simulink model "sarzni_reaktor1_2"  (R2020b)
settings: Solver=VariableStepAuto  StartTime=0.0  StopTime=tSim  RelTol=1e-3
values from neighbouring files (symbols this model uses):
  T_ref = 50    [reactortest.m]
libraries: pid_lib x2, reaktor x1
settings Model: Creator=micha  LastModifiedBy=64220310
settings DebuggingCC: UnconnectedInputMsg=none  UnconnectedOutputMsg=none  UnconnectedLineMsg=none
settings ModelReferenceCC: EnableRefExpFcnMdlSchedulingChecks=off
settings RTWCC: GPUComputeCapability=5.0

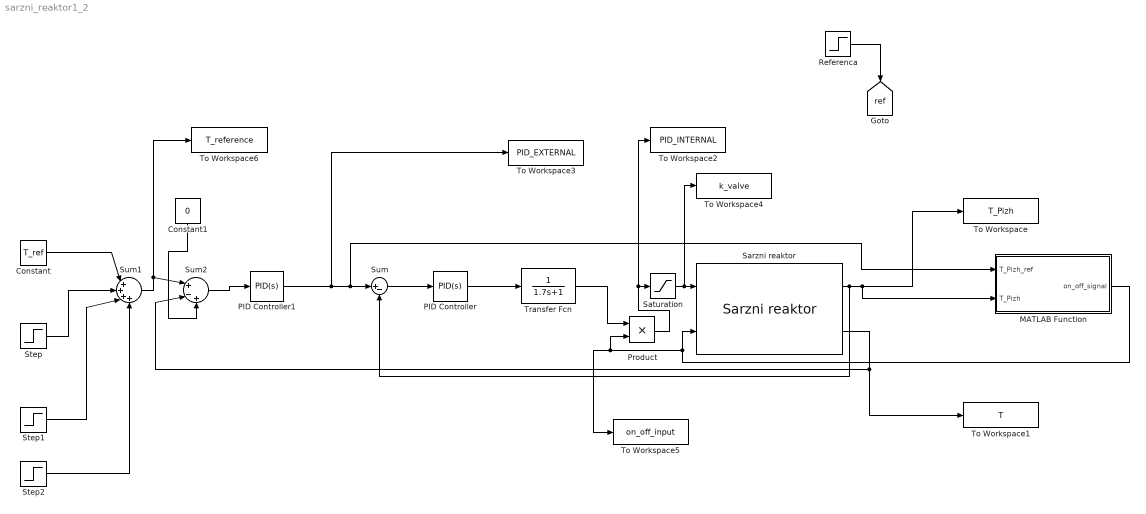
== system sarzni_reaktor1_2 ==
  Constant : Constant  Value=T_ref
  Constant1 : Constant  Value=0
  MATLAB Function : MATLAB Function  AncestorBlock=reaktor/MATLAB Function  TreatAsAtomicUnit=on
  PID Controller : pid_lib/PID Controller  Controller=PID  Form=Parallel  TimeDomain=Continuous-time  UseExternalTs=off  SampleTime=-1  IntegratorMethod=Forward Euler  FilterMethod=Forward Euler  ControllerParametersSource=internal  P=0.22  I=0  D=0  UseFilter=on  N=100  TunerSelectOption=Transfer Function Based (PID Tuner App)  InitialConditionSource=internal  InitialConditionForIntegrator=0  InitialConditionForFilter=0  DifferentiatorICPrevScaledInput=0  ExternalReset=none  TrackingMode=off  Kt=1  LimitOutput=off  SatLimitsSource=internal  UpperSaturationLimit=inf  LowerSaturationLimit=-inf  LinearizeAsGain=on  AntiWindupMode=none  Kb=1  POutMin=[]  POutMax=[]  IOutMin=[]  IOutMax=[]  DOutMin=[]  DOutMax=[]  NOutMin=[]  NOutMax=[]  SumOutMin=[]  SumOutMax=[]  SaturationOutMin=[]  SaturationOutMax=[]  PParamMin=[]  PParamMax=[]  IParamMin=[]  IParamMax=[]  DParamMin=[]  DParamMax=[]  NParamMin=[]  NParamMax=[]  KbParamMin=[]  KbParamMax=[]  KtParamMin=[]  KtParamMax=[]  KbOutMin=[]  KbOutMax=[]  KtOutMin=[]  KtOutMax=[]  IntegratorOutMin=[]  IntegratorOutMax=[]  FilterOutMin=[]  FilterOutMax=[]  SumI1OutMin=[]  SumI1OutMax=[]  SumI2OutMin=[]  SumI2OutMax=[]  SumI3OutMin=[]  SumI3OutMax=[]  SumI4OutMin=[]  SumI4OutMax=[]  SumDOutMin=[]  SumDOutMax=[]  DifferentiatorOutMin=[]  DifferentiatorOutMax=[]  FilterDiffOutCoefMin=[]  FilterDiffOutCoefMax=[]  ReciprocalOutMin=[]  ReciprocalOutMax=[]  SumDenOutMin=[]  SumDenOutMax=[]  SumNumOutMin=[]  SumNumOutMax=[]  DivideOutMin=[]  DivideOutMax=[]  UdiffTsProdOutMin=[]  UdiffTsProdOutMax=[]  NTsProdOutMin=[]  NTsProdOutMax=[]  UintegralTsProdOutMin=[]  UintegralTsProdOutMax=[]  UngainTsProdOutMin=[]  UngainTsProdOutMax=[]  IntegratorContinuousStateAttributes=''  IntegratorStateMustResolveToSignalObject=off  IntegratorRTWStateStorageClass=Auto  FilterContinuousStateAttributes=''  FilterStateMustResolveToSignalObject=off  FilterRTWStateStorageClass=Auto  ParallelPVariant=InternalParameters  IdealPVariant=Disabled  IVariant=InternalParameters  DVariant=InternalParameters  IntegratorVariant=Continuous  SatVariant=Disabled  AWVariant=Passthrough  PCopyVariant=Disabled  TRVariant=Disabled  FdbkBlocksVariant=Forward  IdealPFdbkVariant=Disabled  SatFdbkVariant=Disabled  DerivativeFilterVariant=ContFilter  NVariant=InternalParameters  NCopyVariant=Disabled  FilterICVariant=InternalICsFilter  IntegratorICVariant=InternalICs  ExternalResetVariant=Disabled  TRSumVariant=Passthrough  SumFdbkVariant=Disabled  SumVariant=Sum_PID  TsampFilterVariant=InternalTs  TsampNgainVariant=Passthrough  TsampIntegralVariant=Passthrough  ExternalSaturationOutDataTypeStr=Inherit: Same as second input
  PID Controller1 : pid_lib/PID Controller  Controller=PID  Form=Parallel  TimeDomain=Continuous-time  UseExternalTs=off  SampleTime=-1  IntegratorMethod=Forward Euler  FilterMethod=Forward Euler  ControllerParametersSource=internal  P=10  I=0.001  D=0  UseFilter=on  N=100  TunerSelectOption=Transfer Function Based (PID Tuner App)  InitialConditionSource=internal  InitialConditionForIntegrator=0  InitialConditionForFilter=0  DifferentiatorICPrevScaledInput=0  ExternalReset=none  TrackingMode=off  Kt=1  LimitOutput=on  SatLimitsSource=internal  UpperSaturationLimit=60  LowerSaturationLimit=10  LinearizeAsGain=on  AntiWindupMode=back-calculation  Kb=0.00005  POutMin=[]  POutMax=[]  IOutMin=[]  IOutMax=[]  DOutMin=[]  DOutMax=[]  NOutMin=[]  NOutMax=[]  SumOutMin=[]  SumOutMax=[]  SaturationOutMin=[]  SaturationOutMax=[]  PParamMin=[]  PParamMax=[]  IParamMin=[]  IParamMax=[]  DParamMin=[]  DParamMax=[]  NParamMin=[]  NParamMax=[]  KbParamMin=[]  KbParamMax=[]  KtParamMin=[]  KtParamMax=[]  KbOutMin=[]  KbOutMax=[]  KtOutMin=[]  KtOutMax=[]  IntegratorOutMin=[]  IntegratorOutMax=[]  FilterOutMin=[]  FilterOutMax=[]  SumI1OutMin=[]  SumI1OutMax=[]  SumI2OutMin=[]  SumI2OutMax=[]  SumI3OutMin=[]  SumI3OutMax=[]  SumI4OutMin=[]  SumI4OutMax=[]  SumDOutMin=[]  SumDOutMax=[]  DifferentiatorOutMin=[]  DifferentiatorOutMax=[]  FilterDiffOutCoefMin=[]  FilterDiffOutCoefMax=[]  ReciprocalOutMin=[]  ReciprocalOutMax=[]  SumDenOutMin=[]  SumDenOutMax=[]  SumNumOutMin=[]  SumNumOutMax=[]  DivideOutMin=[]  DivideOutMax=[]  UdiffTsProdOutMin=[]  UdiffTsProdOutMax=[]  NTsProdOutMin=[]  NTsProdOutMax=[]  UintegralTsProdOutMin=[]  UintegralTsProdOutMax=[]  UngainTsProdOutMin=[]  UngainTsProdOutMax=[]  IntegratorContinuousStateAttributes=''  IntegratorStateMustResolveToSignalObject=off  IntegratorRTWStateStorageClass=Auto  FilterContinuousStateAttributes=''  FilterStateMustResolveToSignalObject=off  FilterRTWStateStorageClass=Auto  ParallelPVariant=InternalParameters  IdealPVariant=Disabled  IVariant=InternalParameters  DVariant=InternalParameters  IntegratorVariant=Continuous  SatVariant=Enabled  AWVariant=BackCalculation  PCopyVariant=Disabled  TRVariant=Disabled  FdbkBlocksVariant=Forward  IdealPFdbkVariant=Disabled  SatFdbkVariant=Disabled  DerivativeFilterVariant=ContFilter  NVariant=InternalParameters  NCopyVariant=Disabled  FilterICVariant=InternalICsFilter  IntegratorICVariant=InternalICs  ExternalResetVariant=Disabled  TRSumVariant=Passthrough  SumFdbkVariant=Disabled  SumVariant=Sum_PID  TsampFilterVariant=InternalTs  TsampNgainVariant=Passthrough  TsampIntegralVariant=Passthrough  ExternalSaturationOutDataTypeStr=Inherit: Same as second input
  Product : Product
  Referenca : Step  Time=10000  Before=40  After=45  SampleTime=0
  Sarzni reaktor : reaktor/Sarzni reaktor  anim=1  sum=on
  Saturation : Saturate  UpperLimit=1  LowerLimit=0
  Step : Step  Time=10000  After=-6  SampleTime=1
  Step1 : Step  Time=15000  After=4  SampleTime=1
  Step2 : Step  Time=20000  After=-17  SampleTime=1
  Sum : Sum  Inputs=|+-
  Sum1 : Sum  Inputs=|++++
  Sum2 : Sum  Inputs=|+-+
  To Workspace : ToWorkspace  VariableName=T_Pizh  SaveFormat=Timeseries  SampleTime=-1
  To Workspace1 : ToWorkspace  VariableName=T  SaveFormat=Timeseries  SampleTime=-1
  To Workspace2 : ToWorkspace  VariableName=PID_INTERNAL  SaveFormat=Timeseries  SampleTime=-1
  To Workspace3 : ToWorkspace  VariableName=PID_EXTERNAL  SaveFormat=Timeseries  SampleTime=-1
  To Workspace4 : ToWorkspace  VariableName=k_valve  SaveFormat=Timeseries  SampleTime=-1
  To Workspace5 : ToWorkspace  VariableName=on_off_input  SaveFormat=Timeseries  SampleTime=-1
  To Workspace6 : ToWorkspace  VariableName=T_reference  SaveFormat=Timeseries  SampleTime=-1
  Transfer Fcn : TransferFcn  Denominator=[1.7 1]
  tag scope: ref=global
  wires:
  MATLAB Function/1(on_off_signal) -> Sarzni reaktor/2, Product/2, To Workspace5/1
  Sum/1 -> PID Controller/1
  Referenca/1 -> [ref]
  Sarzni reaktor/2 -> To Workspace1/1, Sum2/2
  Product/1 -> To Workspace2/1, Saturation/1
  Saturation/1 -> To Workspace4/1, Sarzni reaktor/1
  PID Controller1/1 -> Sum/1, MATLAB Function/1(T_Pizh_ref), To Workspace3/1
  Sarzni reaktor/1 -> MATLAB Function/2(T_Pizh), To Workspace/1, Sum/2
  Sum2/1 -> PID Controller1/1
  Step/1 -> Sum1/2
  Constant/1 -> Sum1/1
  Sum1/1 -> To Workspace6/1, Sum2/1
  Step1/1 -> Sum1/3
  Step2/1 -> Sum1/4
  Constant1/1 -> Sum2/3
  PID Controller/1 -> Transfer Fcn/1
  Transfer Fcn/1 -> Product/1

== matlab function sarzni_reaktor1_2/MATLAB Function ==
  settings: updateMethod=DISCRETE  sampleTime=0.01
  data: T_Pizh_ref input; on_off_signal output; T_Pizh input
function on_off_signal = hot_cold_selection_logic_asymmetric(T_Pizh_ref, T_Pizh)
  % Defines the switching signal for hot (1) or cold (-1) water.
  % Implements ASYMMETRIC hysteresis to prevent rapid valve switching.

  persistent current_selection; % Remembers the current valve state: 1 for hot, -1 for cold.

  % --- Asymmetric Hysteresis Offsets (in degrees Celsius) ---
  % These are the key parameters you'll need to tune.
  % Offset when considering switching from HOT to COLD:
  HYSTERESIS_OFFSET_FOR_SWITCHING_TO_COLD = 6; % Example value (e.g., if T_Pizh_ref drops 4C below T_Pizh)
  % Offset when considering switching from COLD to HOT:
  HYSTERESIS_OFFSET_FOR_SWITCHING_TO_HOT  = 6; % Example value (e.g., if T_Pizh_ref rises 6C above T_Pizh)
  
  % --- Initialization: Determine the initial state on the very first call ---
  if isempty(current_selection)
    % Use the system's documented initial jacket temperature (ambient T_O).
    % You had this as 12.0 in your provided code.
    initial_T_Pizh_system_assumption = 12.0; 

    % Decide initial valve selection. For initialization, we can use the
    % respective offsets to determine if a significant heating or cooling
    % action is immediately required from the assumed initial state.
    if T_Pizh_ref > (initial_T_Pizh_system_assumption + HYSTERESIS_OFFSET_FOR_SWITCHING_TO_HOT)
        current_selection = 1;  % Start with HOT water if setpoint is significantly above initial.
    elseif T_Pizh_ref < (initial_T_Pizh_system_assumption - HYSTERESIS_OFFSET_FOR_SWITCHING_TO_COLD)
        current_selection = -1; % Start with COLD water if setpoint is significantly below initial.
    else
        % T_Pizh_ref is relatively close to the initial assumed temperature;
        % make a sensible default choice based on whether heating or cooling is generally needed.
        if T_Pizh_ref > initial_T_Pizh_system_assumption
            current_selection = 1;  % Default to heating if setpoint is above initial.
        else
            current_selection = -1; % Default to cooling if setpoint is at or below initial.
        end
    end
  end

  % --- Main Switching Logic with Asymmetric Hysteresis ---
  % This logic executes on every call after the initialization.

  if current_selection == 1 % Currently supplying HOT water
    % Condition to switch from HOT to COLD:
    % If T_Pizh_ref drops sufficiently below the current T_Pizh,
    % using the specific offset for switching TO COLD.
    if T_Pizh_ref < (T_Pizh - HYSTERESIS_OFFSET_FOR_SWITCHING_TO_COLD)
      current_selection = -1; % Switch to COLD water.
    end
  else % current_selection == -1, currently supplying COLD water
    % Condition to switch from COLD to HOT:
    % If T_Pizh_ref rises sufficiently above the current T_Pizh,
    % using the specific offset for switching TO HOT.
    if T_Pizh_ref > (T_Pizh + HYSTERESIS_OFFSET_FOR_SWITCHING_TO_HOT)
      current_selection = 1;  % Switch to HOT water.
    end
  end

  on_off_signal = current_selection; % Output the determined valve state.
end
